simulink model "IEEE9-WT-PV"  (R2024a)
settings: Solver=FixedStepDiscrete  StartTime=0.0  StopTime=Tend  RelTol=1e-3
values from neighbouring files (symbols this model uses):
  beta_0 = 0    [data_WT.m]
  C_4 = 0.1670*C_b    (= 1.00487241952e-06)    [main.m]
  C_6 = 0.2835*C_b    (= 1.70587623314e-06)    [main.m]
  C_8 = 0.2275*C_b    (= 1.36891302659e-06)    [main.m]
  C_dc = 2*S_LV_base*H_DC_base/V_dc_base^2    (= 0.478267523722)    [data_WT.m]    (also in main.m = 1.6)
  C_f = C_f_pu*C_LV_base    (= 0.001461477898)    [data_WT.m]    (also in main.m = 0.00530516476973)
  f_b = 50    [data_WT.m]    (also in main.m)
  fdr_m = 0.05    [main.m]
  fdr_q = 0.01    [main.m]
  G_diff = ss(c2d(s/(20e-3/3*s+1),T_s_cont,'tustin'))    [data_WT.m]
  G_lowpass_disc = ss(c2d(G_lowpass,T_s_cont,'tustin'))    [data_WT.m]
  G_lowpass_disc_1khz = ss(c2d(G_lowpass_1khz,T_s_cont,'tustin'))    [data_WT.m]
  G_setpoint_lowpass_disc = ss(c2d(ss(1/(0.1*s+1)),T_s_cont,'tustin'))    [main.m]
  G_sm_dis = ss(c2d(G_cont_sm,T_s_sim,'tustin'))    [main.m]
  GSC_theta0 = -45.0572/180*pi*0-60/180*pi    (= -1.0471975512)    [data_WT.m]
  I0_total1 = Npar1*I0    (= 7.7895e-08)    [data_PV.m]
  I_GSC_base = S_GSC_base/V_LV_base    (= 30303.030303)    [data_WT.m]
  I_PMSG_0 = T_park(0)^-1*[Z_PMSG^-1*V_LV_base*sqrt(2/3)*([cos(RSC_theta0);sin(RSC_theta0)]-[cos(PMSG_theta0);sin(PMSG_theta0)]);0]    [data_WT.m]
  IL_total1 = Npar1*IL    (= 50459)    [data_PV.m]
  Ipv_scmax1 = Npar1*Ipv_sc    (= 50300)    [data_PV.m]
  island_q = [-0.1312   -0.0230   -0.0343]    [main.m]
  island_Vdc = [1 1.2853    Vpv_mppmax2/Vdc_n]    [main.m]
  island_Vdc_r = [1 1.3430 1.4716]    [main.m]
  island_Vm = [1 1 1]    [main.m]
  J_PMSG_WT_MS = 2*H_PMSGWT_LS*S_PMSG_base/(2*pi*f_b)^2    (= 630.526507942)    [data_WT.m]
  k_p_GSC = 0.02    [data_WT.m]
  k_p_MSC = k_p_GSC    (= 0.02)    [data_WT.m]
  k_theta_GSC = 0.1    [data_WT.m]
  k_theta_MSC = 2/0.6    (= 3.33333333333)    [data_WT.m]
  K_WT_ff_i = 1    [main.m]
  K_WT_ff_v = 1    [main.m]
  K_WT_i_i = 0.79    [main.m]
  K_WT_i_v = 0.69    [main.m]
  K_WT_p_i = 2.1    [main.m]
  K_WT_p_v = 0.15    [main.m]
  Kff_v = 1    [main.m]
  Kffpv_i = 1    [main.m]
  Kp_beta = 270*0    (= 0)    [data_WT.m]
  Kpvi_i1 = Ki_i*Vpv_m/Ipv_b_LV    [main.m]
  Kpvi_v1 = Ki_v*Ipv_b_LV/Vpv_m    [main.m]
  Kpvp_i1 = Kp_i*Vpv_m/Ipv_b_LV    [main.m]
  Kpvp_v1 = Kp_v*Ipv_b_LV/Vpv_m    [main.m]
  L1_pu = 1*0.0186/m    (= 0.000186)    [main.m]
  L_45 = L_lines(2)    [main.m]
  L_56 = L_lines(3)    [main.m]
  L_67 = L_lines(5)    [main.m]
  L_78 = L_lines(6)    [main.m]
  L_89 = L_lines(8)    [main.m]
  L_94 = L_lines(9)    [main.m]
  L_f = L_f_pu*L_LV_base    (= 3.46639466054e-05)    [data_WT.m]    (also in main.m = 9.54929658551e-06)
  L_PMSG = L_PMSG_PU*L_LV_base    (= 3.46639466054e-05)    [data_WT.m]
  main_p = 0.575    [main.m]
  mpv_dc1 = fdr*kg1*w_b/Vdc_n    [main.m]
  mpv_dc1_r = fdr*kg1_r*w_b/Vdc_n    [main.m]
  mpv_p1 = fdr_p/Vdc_n*w_b    [main.m]
  mpv_q1 = fdr_q*Vpv_m/S_b    [main.m]
  Notch_w_10khz = ss(c2d((s^2+w0_f10khz^2)/(s^2+w0_f10khz/Q_f10khz*s+w0_f10khz^2),T_s_sim,'tustin'))    [data_WT.m]
  omega_base = 2*pi*f_b    (= 314.159265359)    [data_WT.m]    (also in main.m)
  omega_wt = 1.4    [data_WT.m]
  R1_pu = 1*0.00734/m    (= 7.34e-05)    [main.m]
  R_45 = R_lines(2)    [main.m]
  R_56 = R_lines(3)    [main.m]
  R_67 = R_lines(5)    [main.m]
  R_78 = R_lines(6)    [main.m]
  R_89 = R_lines(8)    [main.m]
  R_94 = R_lines(9)    [main.m]
  R_f = R_f_pu*Z_LV_base    (= 0.001089)    [data_WT.m]    (also in main.m = 0.0003)
  R_PMSG = R_PMSG_PU*Z_LV_base    (= 0.005445)    [data_WT.m]
  Rpvs_total1 = Rpv_s*Nser1/Npar1    (= 0.0067482)    [data_PV.m]
  RSC_theta0 = 180/180*pi    (= 3.14159265359)    [data_WT.m]
  Rss1 = Vpv_ocmax1/(IL_total1-I0_total1*(exp(Vpv_ocmax1/VT_total1) -1))    [data_PV.m]
  S_b = 100*(10^6)    (= 100000000)    [main.m]
  S_bt = S_b    (= 100000000)    [main.m]
  S_GSC_base = S_LV_base    (= 100000000)    [data_WT.m]
  S_PMSG_base = S_WTPMSG_base    (= 100000000)    [data_WT.m]
  T_load = 20    [main.m]
  T_pitch_servo = 0.5    [data_WT.m]
  T_redispatch = 25    [main.m]
  T_s_cont = 1e-4    (= 0.0001)    [data_WT.m]
  T_s_sim = 1e-7    (= 1e-07)    [data_WT.m]
  V1_rms = 1000    [main.m]
  V2_rms = 13800    [main.m]
  V_dc_base = 7.92e3    (= 7920)    [data_WT.m]
  V_LV_base = 3.3e3    (= 3300)    [data_WT.m]
  V_m = sqrt(2/3)*V1_rms    [main.m]
  v_wind = 12    [data_WT.m]
  Vdc_n = 3*V_m    [main.m]
  Vpv_mppmax1 = Nser1*Vpv_mpp    (= 2945.7)    [data_PV.m]
  Vpv_ocmax1 = Nser1*Vpv_oc    (= 3671.1)    [data_PV.m]
  VT_total1 = VT*Nser1    (= 135.150894483)    [data_PV.m]
  w_b = 2*pi*f_b    (= 314.159265359)    [data_WT.m]    (also in main.m)
undefined symbols (not defined in the file or in its folder): D1, Delta, DiscIntNeverNeededParam, i_dc, PI_pitch
libraries: spsThreePhaseVIMeasurementLib x15, spsThreePhaseSeriesRLCBranchLib x11, spsabctodq0Lib x8, spsThreePhaseTransformerTwoWindingsLib x5, spsThreePhaseParallelRLCLoadLib x5, spsGroundLib x5, spsSeriesRLCBranchLib x5, spsCurrentMeasurementLib x5, spsVoltageMeasurementLib x4, spsPower3phInstantaneousLib x4, spsdq0toabcLib x4, spsThreePhaseParallelRLCBranchLib x3
(part 3 of 3)

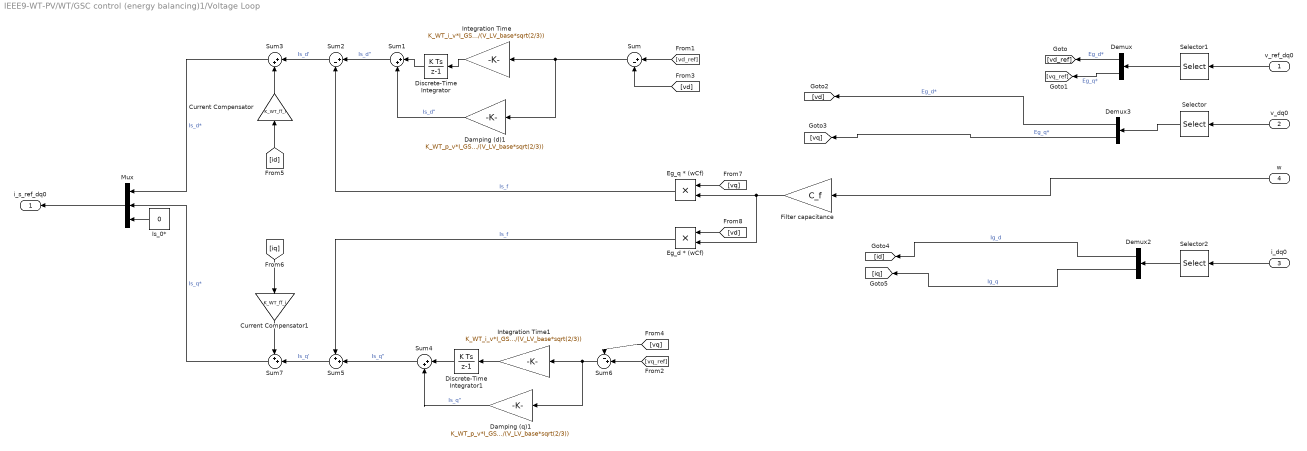
== system IEEE9-WT-PV/WT/GSC control (energy balancing)1/Voltage Loop ==
  v_ref_dq0 : Inport
  v_dq0 : Inport  Port=2
  i_dq0 : Inport  Port=3
  w : Inport  Port=4
  Current Compensator : Gain  Gain=K_WT_ff_i
  Current Compensator1 : Gain  Gain=K_WT_ff_i
  Damping (d)1 : Gain  Gain=K_WT_p_v*I_GSC_base/(V_LV_base*sqrt(2/3))
  Damping (q)1 : Gain  Gain=K_WT_p_v*I_GSC_base/(V_LV_base*sqrt(2/3))
  Demux : Demux  Outputs=2
  Demux2 : Demux  Outputs=2
  Demux3 : Demux  Outputs=2
  Discrete-Time Integrator : DiscreteIntegrator  SampleTime=T_s_cont  ICPrevOutput=DiscIntNeverNeededParam  ICPrevScaledInput=DiscIntNeverNeededParam
  Discrete-Time Integrator1 : DiscreteIntegrator  SampleTime=T_s_cont  ICPrevOutput=DiscIntNeverNeededParam  ICPrevScaledInput=DiscIntNeverNeededParam
  Eg_d * (wCf) : Product  RndMeth=Zero
  "Eg_q * (wCf) " : Product  RndMeth=Zero
  Filter capacitance : Gain  Gain=C_f
  Integration Time : Gain  Gain=K_WT_i_v*I_GSC_base/(V_LV_base*sqrt(2/3))
  Integration Time1 : Gain  Gain=K_WT_i_v*I_GSC_base/(V_LV_base*sqrt(2/3))
  Is_0* : Constant  Value=0  SampleTime=T_s_cont
  Mux : Mux  Inputs=3
  Selector : Selector  InputPortWidth=3  IndexOptions=Index vector (dialog)  Indices=[1 2]  OutputSizes=1
  Selector1 : Selector  InputPortWidth=3  IndexOptions=Index vector (dialog)  Indices=[1 2]  OutputSizes=1
  Selector2 : Selector  InputPortWidth=3  IndexOptions=Index vector (dialog)  Indices=[1 2]  OutputSizes=1
  Sum : Sum  Inputs=|+-
  Sum1 : Sum  Inputs=|++
  Sum2 : Sum  Inputs=|+-
  Sum3 : Sum  Inputs=|++
  Sum4 : Sum  Inputs=|++
  Sum5 : Sum  Inputs=++|
  Sum6 : Sum  Inputs=-+|
  Sum7 : Sum  Inputs=++|
  i_s_ref_dq0 : Outport  VectorParamsAs1DForOutWhenUnconnected=off
  wires:
  Is_0*/1 -> Mux/3
  w/1 -> Filter capacitance/1
  Integration Time1/1 -> Discrete-Time Integrator1/1
  Discrete-Time Integrator1/1 -> Sum4/1
  Eg_d * (wCf)/1 -> Sum5/1  "Is_f"
  Sum7/1 -> Mux/2  "Is_q*"
  Sum2/1 -> Sum3/1  "Is_d'"
  Current Compensator/1 -> Sum3/2
  Current Compensator1/1 -> Sum7/1
  "Eg_q * (wCf) "/1 -> Sum2/2  "Is_f"
  Filter capacitance/1 -> "Eg_q * (wCf) "/2, Eg_d * (wCf)/2
  Sum1/1 -> Sum2/1  "Is_d\""
  Sum5/1 -> Sum7/2  "Is_q'"
  Discrete-Time Integrator/1 -> Sum1/1
  Integration Time/1 -> Discrete-Time Integrator/1
  Sum3/1 -> Mux/1  "Is_d*"
  Sum4/1 -> Sum5/2  "Is_q\""
  Selector/1 -> Demux3/1
  Selector1/1 -> Demux/1
  Selector2/1 -> Demux2/1
  Mux/1 -> i_s_ref_dq0/1
  Sum/1 -> Damping (d)1/1, Integration Time/1
  Sum6/1 -> Damping (q)1/1, Integration Time1/1
  Demux/1 -> [vd_ref]  "Eg_d*"
  Demux/2 -> [vq_ref]  "Eg_q*"
  Demux3/1 -> [vd]  "Eg_d*"
  Demux3/2 -> [vq]  "Eg_q*"
  [vd_ref] -> Sum/1
  [vq_ref] -> Sum6/2
  [vd] -> Sum/2
  [vq] -> Sum6/1
  Damping (q)1/1 -> Sum4/2  "Is_q\""
  Demux2/1 -> [id]  "Ig_d"
  Demux2/2 -> [iq]  "Ig_q"
  [id] -> Current Compensator/1
  [iq] -> Current Compensator1/1
  Damping (d)1/1 -> Sum1/2  "Is_d\""
  [vd] -> Eg_d * (wCf)/1
  [vq] -> "Eg_q * (wCf) "/1
  v_ref_dq0/1 -> Selector1/1
  v_dq0/1 -> Selector/1
  i_dq0/1 -> Selector2/1

== system IEEE9-WT-PV/WT/MSC control1/dc voltage saturation ==
  w_max : Inport
  w_measurement : Inport  Port=2
  w_mpp : Inport  Port=3
  Discrete-Time Integrator1 : DiscreteIntegrator  SampleTime=T_s_cont  LimitOutput=on  UpperSaturationLimit=0  ICPrevOutput=DiscIntNeverNeededParam  ICPrevScaledInput=DiscIntNeverNeededParam
  Discrete-Time Integrator2 : DiscreteIntegrator  SampleTime=T_s_cont  LimitOutput=on  LowerSaturationLimit=0  ICPrevOutput=DiscIntNeverNeededParam  ICPrevScaledInput=DiscIntNeverNeededParam
  Gain1 : Gain  Gain=0.63
  Gain2 : Gain  Gain=0.09
  Gain5 : Gain  Gain=0.73
  Gain7 : Gain  Gain=0.03
  Gain8 : Gain  Gain=2*pi*f_b
  Saturation1 : Saturate  UpperLimit=inf  LowerLimit=0
  Saturation2 : Saturate  UpperLimit=0  LowerLimit=-inf
  Sum10 : Sum  Inputs=|++
  Sum11 : Sum  Inputs=|++
  Sum12 : Sum  Inputs=+-
  Sum17 : Sum  Inputs=+|-
  Sum8 : Sum  Inputs=-+
  w : Outport
  wires:
  Sum11/1 -> Sum17/2
  w_max/1 -> Sum8/1
  Sum8/1 -> Gain2/1, Gain7/1
  Saturation2/1 -> Sum11/1
  w_measurement/1 -> Sum12/1, Sum8/2
  Gain5/1 -> Saturation2/1
  Discrete-Time Integrator2/1 -> Sum10/2
  Saturation1/1 -> Sum10/1
  Sum10/1 -> Sum17/1
  Sum12/1 -> Gain5/1, Gain1/1
  Gain1/1 -> Discrete-Time Integrator1/1
  Gain7/1 -> Saturation1/1
  Discrete-Time Integrator1/1 -> Sum11/2
  Gain2/1 -> Discrete-Time Integrator2/1
  Sum17/1 -> Gain8/1
  w_mpp/1 -> Sum12/2
  Gain8/1 -> w/1
